simulink model "GreenhousePlantWithControl"  (R2023b)
settings: Solver=VariableStepAuto  StartTime=0.0  StopTime=1e8  RelTol=1e-3
model workspace (MAT data in the model file):
  CFM2MS = Simulink.Parameter
  CFM2MS.Value = 0.00047194745
  CFM2MS.DataType = 'auto'
  CFM2MS.Complexity = 'real'
  CFM2MS.Dimensions = [1 1]
  Cp = Simulink.Parameter
  Cp.Value = 1005
  Cp.DataType = 'auto'
  Cp.DocUnits = 'J/(kg*K)'
  Cp.Complexity = 'real'
  Cp.Dimensions = [1 1]
  Density = Simulink.Parameter
  Density.Value = 1.225
  Density.DataType = 'auto'
  Density.DocUnits = 'kg/m^3'
  Density.Complexity = 'real'
  Density.Dimensions = [1 1]
  Height = Simulink.Parameter
  Height.Value = 3
  Height.DataType = 'auto'
  Height.DocUnits = 'm'
  Height.Complexity = 'real'
  Height.Dimensions = [1 1]
  Length = Simulink.Parameter
  Length.Value = 5
  Length.DataType = 'auto'
  Length.DocUnits = 'm'
  Length.Complexity = 'real'
  Length.Dimensions = [1 1]
libraries: fl_lib x7, nesl_utility x5, SignalEditorBlockLib x1
settings Model: Creator=vboutrou  LastModifiedBy=vboutrou
settings RTWCC: Toolchain=MinGW64 | CMake/gmake (64-bit Windows)  BuildConfiguration=Release
settings SimscapeCC: SimscapeLogType=all  SimscapeLogLimitData=off

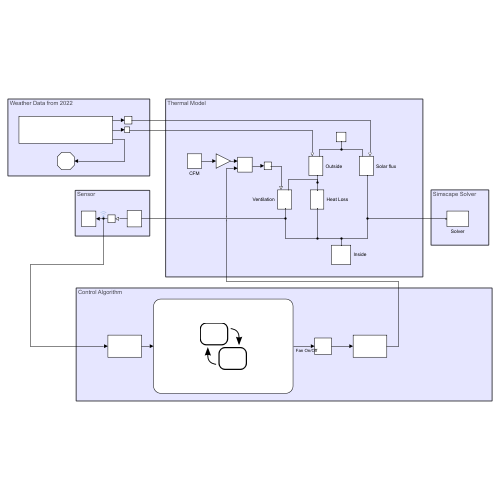
[thumbnail: Simulink's stored preview of the top-level diagram]
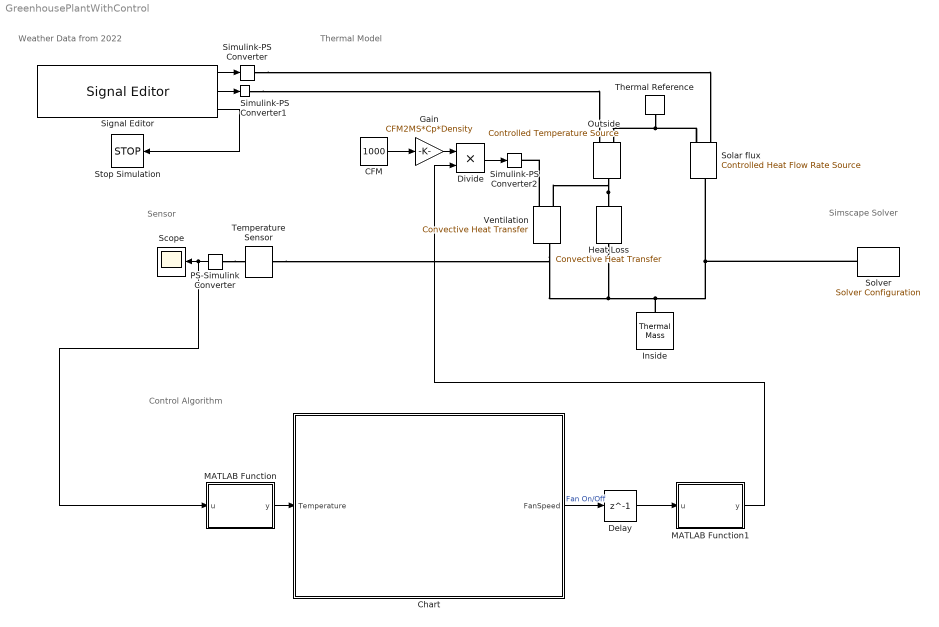
== system GreenhousePlantWithControl ==
  note: Simscape Solver
  note: Sensor
  note: Thermal Model
  note: Weather Data from 2022
  note: Control Algorithm
  CFM : Constant  Value=1000
  Chart : Stateflow chart  TreatAsAtomicUnit=on
  Delay : Delay  DelayLength=1
  Divide : Product  Inputs=**
  Gain : Gain  Gain=CFM2MS*Cp*Density
  Heat Loss : fl_lib/Thermal/Thermal Elements/Convective Heat Transfer  thermal_type=foundation.enum.constant_variable.constant  area=Length^2+4*Length*Height m^2  heat_tr_coeff=10 W/(K*m^2)  min_heat_tr_coeff=1e-3 W/(K*m^2)  T_specify=off  T_priority=None  T=0 K  T_nominal_specify=off  T_nominal_unit=K  T_nominal_value=1  Q_specify=off  Q_priority=None  Q=0 W  Q_nominal_specify=off  Q_nominal_unit=W  Q_nominal_value=1
  Inside : fl_lib/Thermal/Thermal Elements/Thermal Mass  mass_type=foundation.enum.constant_variable.constant  mass=Density*(Height*Length)*Length kg  sp_heat=1005 J/(K*kg)  mass_min=1e-6 kg  num_ports=foundation.enum.numPorts2.one  m_specify=off  m_priority=High  m=1 kg  m_nominal_specify=off  m_nominal_unit=kg  m_nominal_value=1  T_specify=off  T_priority=High  T=300 K  T_nominal_specify=off  T_nominal_unit=K  T_nominal_value=1  Q_specify=off  Q_priority=None  Q=0 W  Q_nominal_specify=off  Q_nominal_unit=W  Q_nominal_value=1
  MATLAB Function : MATLAB Function  TreatAsAtomicUnit=on
  MATLAB Function1 : MATLAB Function  TreatAsAtomicUnit=on
  Outside : fl_lib/Thermal/Thermal Sources/Controlled Temperature Source
  PS-Simulink Converter : nesl_utility/PS-Simulink Converter  PhysicalDomain=network_engine_domain  SubClassName=ps_output  LeftPortType=input  RightPortType=output  PseudoPeriodic=off  Frequencies=[]  VectorFormat=inherit  Unit=inherit  AffineConversion=off
  Scope : Scope
  Signal Editor : SignalEditorBlockLib/Signal Editor  FileName=Weather2022.mat  ActiveScenario=Weather2022  ActiveSignal=SolarFlux  IsBus=off  OutputBusObjectStr=Bus: BusObject  SampleTime=0  ZeroCross=off  OutputAfterFinalValue=Setting to zero  Unit=inherit  PreserveSignalName=on  ApplySigPropsToAllScenarios=on  ApplySigPropsToAllSignals=on
  Simulink-PS Converter : nesl_utility/Simulink-PS Converter  PhysicalDomain=network_engine_domain  SubClassName=ps_input  LeftPortType=input  RightPortType=output  PseudoPeriodic=off  Frequencies=[]  NoiseDistribution=none  NoiseParameters=[]  Unit=W  AffineConversion=off  FilteringAndDerivatives=provide  SimscapeFilterOrder=1  InputFilterTimeConstant=0.001  UdotUserProvided=0
  Simulink-PS Converter1 : nesl_utility/Simulink-PS Converter  PhysicalDomain=network_engine_domain  SubClassName=ps_input  LeftPortType=input  RightPortType=output  PseudoPeriodic=off  Frequencies=[]  NoiseDistribution=none  NoiseParameters=[]  Unit=K  AffineConversion=off  FilteringAndDerivatives=provide  SimscapeFilterOrder=1  InputFilterTimeConstant=0.001  UdotUserProvided=0
  Simulink-PS Converter2 : nesl_utility/Simulink-PS Converter  PhysicalDomain=network_engine_domain  SubClassName=ps_input  LeftPortType=input  RightPortType=output  PseudoPeriodic=off  Frequencies=[]  NoiseDistribution=none  NoiseParameters=[]  Unit=W/(K*m^2)  AffineConversion=off  FilteringAndDerivatives=provide  SimscapeFilterOrder=1  InputFilterTimeConstant=0.001  UdotUserProvided=0
  Solar flux : fl_lib/Thermal/Thermal Sources/Controlled Heat Flow Rate Source
  Solver : nesl_utility/Solver Configuration  PhysicalDomain=network_engine_domain  SubClassName=solver  LeftPortType=input  RightPortType=generic  Tones=[]  Harmonics=[]  SimulateNoise=off  Profile=off  UseLocalSampling=off  EnableSwitchedLinearOptims=on  FrequencyDomain=off  UseCCode=off  RelTol=0.001  AbsTol=0.001  MinStep=1e-09  ToWorkspace=off  RevertToSquareIcSolve=off  NumHomotopyIterations=100  PhasorMode=off  PhasorModeNumHarmonics=1  ConsistencySolver=NEWTON_XTOL_AFTER_FTOL  IndexReductionMethod=DerivativeReplacement  DoDC=on  ResidualTolerance=1e-09  ConsistencyTolSource=GLOBAL  ConsistencyAbsTol=0.001  ConsistencyRelTol=0.001  ConsistencyTolFactor=0.001  UseLocalSolver=off  LocalSolverChoice=NE_BACKWARD_EULER_ADVANCER  ResolveIndetEquations=on  FunctionEvalNumThread=1  LocalSolverSampleTime=0.001  DoFixedCost=off  MaxNonlinIter=3  MaxModeIter=2  ComputeImpulses=off  ImpulseIterations=2  LinearAlgebra=auto  LinearAlgebraNumThread=0  EquationFormulation=NE_TIME_EF  DelaysMemoryBudget=1024  AutomaticFiltering=on  FilteringTimeConstant=0.001  PartitionStorageMethod=AS_NEEDED  PartitionMemoryBudget=1024  PartitionMethod=ROBUST  MultibodyUseLocalSolver=off  MultibodyLocalSolverChoice=ODE1  MultibodyLocalSolverSampleTime=0.001
  Stop Simulation : Stop
  Temperature Sensor : fl_lib/Thermal/Thermal Sensors/Temperature Sensor  temperature_measure=foundation.enum.MeasurementReference.absolute
      settings: InternalSimscapePortConfiguration="{\"Bottom\":[],\"Left\":[{\"id\":\"A\",\"label\":\"A\",\"type\":\"foundation.thermal.thermal\"}],\"Right\":[{\"id\":\"T\",\"label\":\"T\",\"type\":\"output\"}],\"Top\":[]}"
  Thermal Reference : fl_lib/Thermal/Thermal Elements/Thermal Reference
  Ventilation : fl_lib/Thermal/Thermal Elements/Convective Heat Transfer  thermal_type=foundation.enum.constant_variable.variable  area=1 m^2  heat_tr_coeff=20 W/(K*m^2)  min_heat_tr_coeff=1e-12 W/(K*m^2)  T_specify=off  T_priority=None  T=0 K  T_nominal_specify=off  T_nominal_unit=K  T_nominal_value=1  Q_specify=off  Q_priority=None  Q=0 W  Q_nominal_specify=off  Q_nominal_unit=W  Q_nominal_value=1
      settings: InternalSimscapePortConfiguration="{\"Bottom\":[],\"Left\":[{\"id\":\"A\",\"label\":\"A\",\"type\":\"foundation.thermal.thermal\"},{\"id\":\"var_heat_tr_coeff\",\"label\":\"K\",\"type\":\"input\"}],\"Right\":[{\"id\":\"B\",\"label\":\"B\",\"type\":\"foundation.thermal.thermal\"}],\"Top\":[]}"
  wires:
  Signal Editor/1 -> Simulink-PS Converter/1
  CFM/1 -> Gain/1
  PS-Simulink Converter/1 -> MATLAB Function/1(u), Scope/1
  MATLAB Function/1(y) -> Chart/1(Temperature)
  Signal Editor/3 -> Stop Simulation/1
  Signal Editor/2 -> Simulink-PS Converter1/1
  Chart/1(FanSpeed) -> Delay/1  "Fan On/Off"
  Delay/1 -> MATLAB Function1/1(u)
  Gain/1 -> Divide/1
  Divide/1 -> Simulink-PS Converter2/1
  MATLAB Function1/1(y) -> Divide/2
  connections:
  Simulink-PS Converter1/RConn1 -- Outside/RConn1
  Thermal Reference/LConn1 -- Solar flux/RConn2 -- Outside/RConn2
  Inside/LConn1 -- Temperature Sensor/LConn1 -- Ventilation/RConn1 -- Heat Loss/LConn1 -- Solver/RConn1 -- Solar flux/LConn1
  Outside/LConn1 -- Ventilation/LConn1 -- Heat Loss/RConn1
  Simulink-PS Converter/RConn1 -- Solar flux/RConn1
  Ventilation/LConn2 -- Simulink-PS Converter2/RConn1
  PS-Simulink Converter/LConn1 -- Temperature Sensor/RConn1

== matlab function GreenhousePlantWithControl/MATLAB Function1 ==
  data: u input; y output
function y = fcn(u)
if u == 0
    y = 1e-9;
else
    y = 1;
end

== matlab function GreenhousePlantWithControl/MATLAB Function ==
  data: u input; y output
function y = KelvinToFarenheit(u)

y = (u-273.15)*9/5+32;
end

== stateflow chart GreenhousePlantWithControl/Chart ==
  state InitialState
    FanSpeed = 0;
  state ActivatedState
    FanSpeed = 255;
  (default) -> InitialState
  ActivatedState -> InitialState : [Temperature<= 75]
  InitialState -> ActivatedState : [Temperature >= 80]
  data: Temperature input; FanSpeed output
